simulink model "newtons_cradle"  (R2013b)
settings: Solver=ode45  SolverMode=SingleTasking  StartTime=0.0  StopTime=5  RelTol=1e-3
settings Model: Creator=The MathWorks Inc.  LastModifiedBy=Daniel
settings DataIOCC: SignalLoggingSaveFormat=ModelDataLogs
settings OptimizationCC: BlockReduction=off  BooleanDataType=off  ExpressionDepthLimit=2147483647  InitFltsAndDblsToZero=on
settings DebuggingCC: SignalResolutionControl=TryResolveAllWithWarning  SolverPrmCheckMsg=none  FcnCallInpInsideContextMsg=UseLocalSettings  StateNameClashWarn=warning
settings HardwareCC: TargetUnknown=on
settings SFSimCC: SFSimEnableDebug=off  SFSimOverflowDetection=off  SFSimEcho=off  SimParseCustomCode=off
settings GRTTargetCC: TargetFcnLib=ansi_tfl_tmw_new.mat  CombineOutputUpdateFcns=off  GRTInterface=on

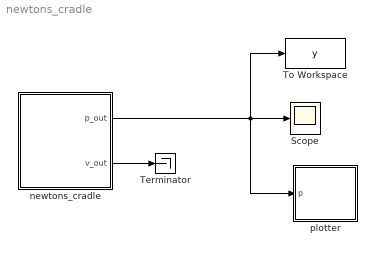
== system newtons_cradle ==
  Scope : Scope
      settings: YMin=-0.75  YMax=0.75
  Terminator : Terminator
  To Workspace : ToWorkspace  VariableName=y  SampleTime=-1
  newtons_cradle : Stateflow chart  TreatAsAtomicUnit=on
  plotter : Stateflow chart  TreatAsAtomicUnit=on
  wires:
  newtons_cradle/1(p_out) -> Scope/1, To Workspace/1, plotter/1(p)
  newtons_cradle/2(v_out) -> Terminator/1

== stateflow chart newtons_cradle/newtons_cradle ==
  settings: updateMethod=CONTINUOUS  executeAtInitialization=1  initializeOutput=1
  state FreeDynamics
    du:
    p_out = p;
    v_out = v;
    p_dot = v;
    v_dot = -g/l*sin(p);
  state resetPositionsAndVelocities [function]
    (default) -> (junction 22) : {i=0;}
    (junction 22) -> (junction 24) [order 1] : [i < k-1]
    (junction 17) -> (junction 22) : {i++;}
    (junction 24) -> (junction 17) [order 2]
    (junction 24) -> (junction 17) [order 1] : // if balls i and i+1
        | // have crossed paths
        | [p[i] < p[i+1]]
        | {
        | // swap positions
        | tmp = p[i];
        | p[i] = p[i+1];
        | p[i+1] = tmp;
        | // swap velocities
        | tmp = v[i];
        | v[i] = v[i+1];
        | v[i+1] = tmp;
        | }
    (junction 22) -> (junction 23) [order 2]
  state collision = isCollisionPossible [function]
    (default) -> (junction 18) : {i=0;}
    (junction 18) -> (junction 20) [order 1] : [i < k-1]
    (junction 20) -> (junction 18) [order 2] : {i++;}
    (junction 18) -> (junction 19) [order 2] : {
        | collision = 0;
        | }
    (junction 20) -> (junction 21) [order 1] : [p[i] < p[i+1]]
        | {
        | collision = 1;
        | }
  (default) -> FreeDynamics : {
      | p = 0;
      | v = 0;
      | p[0] = pi/8;
      | }
  FreeDynamics -> FreeDynamics : [isCollisionPossible()]
      | { resetPositionsAndVelocities(); }
  data: i temporary double; tmp temporary double; collision function_output double; i temporary double; p_out output double size=k; v_out output double size=k; g constant double =9.81; l constant double =1; pi constant double =3.141; p local double size=k; v local double size=k; k constant int32 =3
  data p settings: updateMethod=SF_CONTINUOUS_TIME_DATA
  data v settings: updateMethod=SF_CONTINUOUS_TIME_DATA

== stateflow chart newtons_cradle/plotter ==
  settings: updateMethod=DISCRETE  sampleTime=0.1
  state A
    du:
    ml.sf_newtons_cradle_plotter(p);
  data: p input double
